simulink model "karlman_lanefit"  (R2016a)
settings: Solver=FixedStepDiscrete  StartTime=0.0  StopTime=55  FixedStep=0.1  MaxStep=0.1  RelTol=1e-3
settings Model: Creator=yesimeng  LastModifiedBy=yesimeng

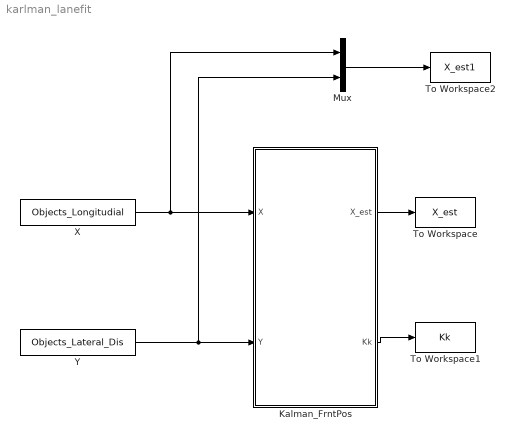
== system karlman_lanefit ==
  Kalman_FrntPos : MATLAB Function  TreatAsAtomicUnit=on
  Mux : Mux  Inputs=2
  To Workspace : ToWorkspace  VariableName=X_est  SampleTime=-1
      settings: Save2DSignal=2-D array (concatenate along first dimension)
  To Workspace1 : ToWorkspace  VariableName=Kk  SampleTime=-1
      settings: Save2DSignal=2-D array (concatenate along first dimension)
  To Workspace2 : ToWorkspace  VariableName=X_est1  SampleTime=-1
      settings: Save2DSignal=2-D array (concatenate along first dimension)
  X : FromWorkspace  VariableName=Objects_Longitudial  SampleTime=0.1
  Y : FromWorkspace  VariableName=Objects_Lateral_Dis  SampleTime=0.1
  wires:
  Y/1 -> Mux/2, Kalman_FrntPos/2(Y)
  X/1 -> Mux/1, Kalman_FrntPos/1(X)
  Kalman_FrntPos/1(X_est) -> To Workspace/1
  Kalman_FrntPos/2(Kk) -> To Workspace1/1
  Mux/1 -> To Workspace2/1

== matlab function karlman_lanefit/Kalman_FrntPos ==
  data: X input; Y input; X_est output; Kk output
function [X_est,Kk] = Kalman_FrntPos(X,Y)
%#codegen
%%
Ts = 0.1;
persistent x_hat Pk 
if isempty(x_hat)
    x_hat = [X,Y,0,0]';        % 最优值初始化
end
if isempty(Pk)
    Pk = eye(4);                   % 最优值误差方差
end
Z = [X;Y];
% Qk = diag([0; 0; 0.33; 0.7])^2;   % 系统误差方差
% Rk = diag([0.18; 0.20])^2;              % 测量误差方差
Qk = diag([0; 0; 0.33; 0.7])^2;   % 系统误差方差
Rk = 10.*diag([0.18; 0.20])^2;              % 测量误差方差
% Qk = diag([0; 0; 0.5; 0.5])^2;   % 系统误差方差
% Rk = 4.*diag([0.5; 0.5])^2;              % 测量误差方差
% Pkk_1 = 10*eye(4);                    % 估测误差方差，上次最优值方差+系统误差方差
% X_est = zeros(len,4);              % 最优值集合
% x_forecast = zeros(5,1);           % 预测值
% z = zeros(4,1);
% 1 状态预测
Ang = atan(x_hat(2)./x_hat(1));
x  = x_hat(1) + x_hat(3).*cos(Ang).*Ts - x_hat(4).*sin(Ang).*Ts;
y  = x_hat(2) + x_hat(3).*sin(Ang).*Ts + x_hat(4).*cos(Ang).*Ts;
vfx = x_hat(3);
vfy = x_hat(4);
% vm  = x_hat(5);
% if isempty(x_forecast)
%     x_forecast = x_hat;        %预测值
% else
    x_forecast = [x; y; vfx; vfy];        %预测值
% end
% 2  观测预测
xg = x;
yg = y;
y_forecast = [xg;yg];
% y_forecast = x_forecast(1:2);
%  状态矩阵
F = zeros(4,4);   % 系统状态方程的雅可比矩阵
F(1,1) =  1;
F(1,3) =  Ts.*cos(Ang);
F(1,4) = -Ts.*sin(Ang);
F(2,2) =  1;
F(2,3) =  Ts.*sin(Ang);
F(2,4) =  Ts.*cos(Ang);
F(3,3) =  1;
F(4,4) =  1;

% temp_sin = sin(atan(y./x));
% temp_cos = cos(atan(y./x));
% temp_sinr = temp_sin ./ (x.^2 + y.^2);
% temp_cosr = temp_cos ./ (x.^2 + y.^2);
% F(1,1) =  vfx*Ts.*y.*temp_sinr + vfy.*Ts.*y.*temp_cosr + 1;
% F(1,2) = -(vfx*Ts.*x.*temp_sinr + vfy.*Ts.*x.*temp_cosr);
% F(1,3) =  temp_cos .* Ts;
% F(1,4) = -temp_sin .* Ts;
% F(2,1) = -vfx*Ts.*y.*temp_cosr + vfy.*Ts.*y.*temp_sinr;
% F(2,2) =  vfx*Ts.*x.*temp_cosr - vfy.*Ts.*x.*temp_sinr + 1;
% F(2,3) =  temp_sin .* Ts;
% F(2,4) =  temp_cos .* Ts;
% F(3,3) = 1;
% F(4,4) = 1;
Pkk_1 = F*Pk*F'+Qk;  %由上次的误差协方差Pk和预测系统误差方差Qk,得出这次预测的误差方差Pkk_1
% 观测矩阵
H = zeros(2,4);
H(1,1) = 1;
H(2,2) = 1;

Kk = Pkk_1*H'*(H*Pkk_1*H'+Rk)^-1;       % 根据这次估计的误差和测量误差，计算增益
x_hat = x_forecast+Kk*(Z-y_forecast);      %校正
Pk = (eye(4)-Kk*H)*Pkk_1;
X_est = x_hat;
